simulink library "library"  (R2020b)
settings: Solver=VariableStepAuto  StartTime=0.0  StopTime=10.0  RelTol=1e-3
undefined symbols (not defined in the file): constants, orbit, sensors, spacecraft
libraries: vrlib x6, cstblocks x1, $bdroot x1
settings Model: Creator=loren  LastModifiedBy=loren

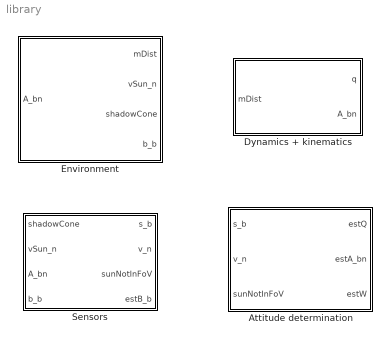
== system library ==
  Attitude determination : Subsystem
  Dynamics + kinematics : Subsystem
  Environment : Subsystem
  Sensors : Subsystem

== system library/Attitude determination ==
  s_b : Inport
  v_n : Inport  Port=2
  sunNotInFoV : Inport  Port=3
  Angular velocity estimation : Subsystem
  DCM : $bdroot/Kinematics/DCM  SystemSampleTime=-1  VariantActivationTime=update diagram  Latency=0  AutoFrameSizeCalculation=off
  MATLAB Function : MATLAB Function  TreatAsAtomicUnit=on
  Memory : Memory  InitialCondition=spacecraft.q0
  estQ : Outport
  estA_bn : Outport  Port=2
  estW : Outport  Port=3
  wires:
  s_b/1 -> MATLAB Function/1(s_b)
  v_n/1 -> MATLAB Function/2(v_n)
  sunNotInFoV/1 -> MATLAB Function/3(sunNotInFoV)
  DCM/1 -> estA_bn/1
  Angular velocity estimation/1(estW) -> estW/1
  MATLAB Function/1(estQ) -> Memory/1, estQ/1, DCM/1, Angular velocity estimation/1(estQ)
  Memory/1 -> MATLAB Function/4(q_old)

== system library/Dynamics + kinematics ==
  mDist : Inport
  Euler eqns. : Subsystem
  Kinematics : Subsystem
  q : Outport
  A_bn : Outport  Port=2
  wires:
  mDist/1 -> Euler eqns./1(mDist)
  Euler eqns./1(w) -> Kinematics/1(w)
  Kinematics/1(q) -> q/1
  Kinematics/2(A_bn) -> A_bn/1

== system library/Environment ==
  A_bn : Inport
  Disturbances : Subsystem
  Orbit propagator : Subsystem
  mDist : Outport
  vSun_n : Outport  Port=2
  shadowCone : Outport  Port=3
  b_b : Outport  Port=4
  wires:
  A_bn/1 -> Disturbances/3(A_bn), Orbit propagator/1(A_bn)
  Orbit propagator/1(rrSc_n) -> Disturbances/1(rrSc_n)
  Orbit propagator/2(vvSc_n) -> Disturbances/2(vvSc_n)
  Orbit propagator/3(A_bl) -> Disturbances/4(A_bl)
  Disturbances/1(mDist) -> mDist/1
  Disturbances/2(vSun_n) -> vSun_n/1
  Disturbances/3(shadowCone) -> shadowCone/1
  Disturbances/4(b_b) -> b_b/1

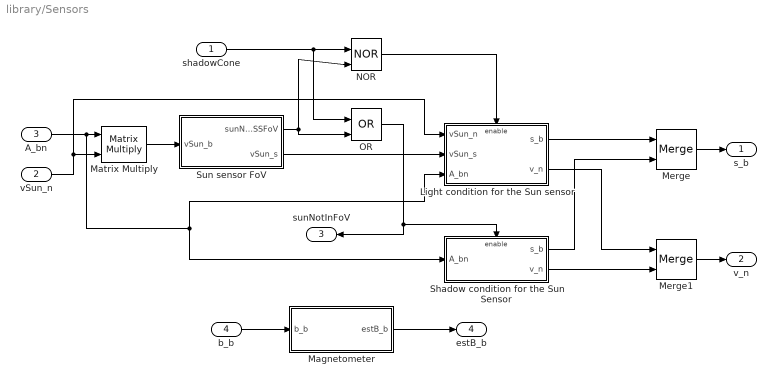
== system library/Sensors ==
  shadowCone : Inport
  vSun_n : Inport  Port=2
  A_bn : Inport  Port=3
  b_b : Inport  Port=4
  Light condition for the Sun sensor : Subsystem  TreatAsAtomicUnit=on
  Magnetometer : Subsystem
  Matrix Multiply : Product  Multiplication=Matrix(*)
  Merge : Merge
  Merge1 : Merge
  NOR : Logic  Operator=NOR  IconShape=distinctive  AllPortsSameDT=off  OutDataTypeStr=boolean
  OR : Logic  Operator=OR  IconShape=distinctive  AllPortsSameDT=off  OutDataTypeStr=boolean
  Shadow condition for the Sun Sensor : Subsystem  TreatAsAtomicUnit=on
  Sun sensor FoV : Subsystem
  s_b : Outport
  v_n : Outport  Port=2
  sunNotInFoV : Outport  Port=3
  estB_b : Outport  Port=4
  wires:
  Sun sensor FoV/1(sunNotInSSFoV) -> OR/2, NOR/2
  shadowCone/1 -> NOR/1, OR/1
  Matrix Multiply/1 -> Sun sensor FoV/1(vSun_b)
  vSun_n/1 -> Light condition for the Sun sensor/1(vSun_n), Matrix Multiply/2
  A_bn/1 -> Shadow condition for the Sun Sensor/1(A_bn), Light condition for the Sun sensor/3(A_bn), Matrix Multiply/1
  Merge/1 -> s_b/1
  Merge1/1 -> v_n/1
  OR/1 -> Shadow condition for the Sun Sensor/Enable, sunNotInFoV/1
  Sun sensor FoV/2(vSun_s) -> Light condition for the Sun sensor/2(vSun_s)
  Light condition for the Sun sensor/1(s_b) -> Merge/1
  Shadow condition for the Sun Sensor/1(s_b) -> Merge/2
  Shadow condition for the Sun Sensor/2(v_n) -> Merge1/2
  Light condition for the Sun sensor/2(v_n) -> Merge1/1
  NOR/1 -> Light condition for the Sun sensor/Enable
  b_b/1 -> Magnetometer/1(b_b)
  Magnetometer/1(estB_b) -> estB_b/1

== system library/Attitude determination/Angular velocity estimation ==
  estQ : Inport
  Constant : Constant
  Derivative : Derivative  CoefficientInTFapproximation=1/100
  Gain : Gain  Gain=2
  MATLAB Function : MATLAB Function  TreatAsAtomicUnit=on
  Matrix Multiply : Product  Multiplication=Matrix(*)
  Varying Lowpass Filter : cstblocks/Linear Parameter Varying/Varying Lowpass Filter  N=2
  estW : Outport
  wires:
  estQ/1 -> Varying Lowpass Filter/1, MATLAB Function/1(q)
  MATLAB Function/1(pinvQ) -> Matrix Multiply/1
  Derivative/1 -> Matrix Multiply/2  "dotQest"
  Matrix Multiply/1 -> Gain/1
  Gain/1 -> estW/1
  Varying Lowpass Filter/1 -> Derivative/1
  Constant/1 -> Varying Lowpass Filter/2

== system library/Dynamics + kinematics/Euler eqns. ==
  mDist : Inport
  Add : Sum  Inputs=-+
  Constant : Constant  Value=spacecraft.I
  Cross Product : vrlib/Utilities/Cross Product
  Gain : Gain  Gain=spacecraft.invI  Multiplication=Matrix(K*u) (u vector)
  Integrator : Integrator  InitialCondition=spacecraft.w0
  Product : Product  Multiplication=Matrix(*)
  w : Outport
  wires:
  Constant/1 -> Product/1
  Integrator/1 -> w/1, Product/2, Cross Product/2  "w"
  Product/1 -> Cross Product/1
  mDist/1 -> Add/2
  Cross Product/1 -> Add/1
  Add/1 -> Gain/1
  Gain/1 -> Integrator/1

== system library/Dynamics + kinematics/Kinematics ==
  w : Inport
  DCM : Subsystem
  Quaternion integration : Subsystem
  q : Outport
  A_bn : Outport  Port=2
  wires:
  w/1 -> Quaternion integration/1(w)
  Quaternion integration/1(q) -> q/1, DCM/1(q)
  DCM/1(A_bn) -> A_bn/1

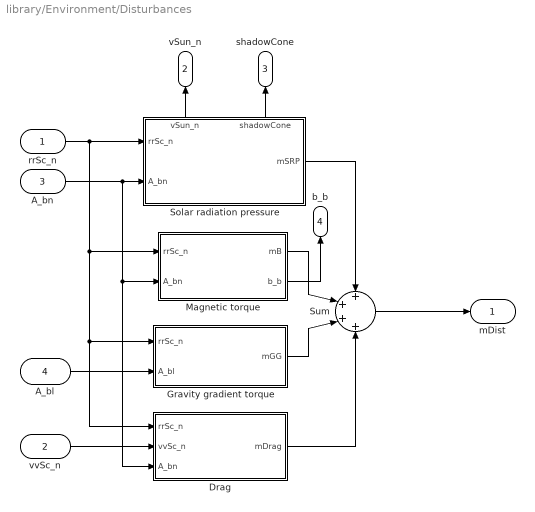
== system library/Environment/Disturbances ==
  rrSc_n : Inport
  vvSc_n : Inport  Port=2
  A_bn : Inport  Port=3
  A_bl : Inport  Port=4
  Drag : Subsystem
  Gravity gradient torque : Subsystem
  Magnetic torque : Subsystem
  Solar radiation pressure : Subsystem
      settings: PortSchema="{\"entries\":[{\"content\":{\"sides\":[{\"content\":{\"connectorIds\":[\"In1\",\"In2\"]},\"type\":\"ConnectorPlacement.EquallySpacedRectSide\",\"uuid\":\"1c58e148-737e-4c26-8467-bf4a1427bac3\"},{\"content\":{\"connectorIds\":[\"Out1\"],\"side\":\"RIGHT\"},\"type\":\"ConnectorPlacement.EquallySpacedRectSide\",\"uuid\":\"1132a1c1-392d-4550-8b40-4ae647f3a6c1\"},{\"content\":{\"connectorIds\":[\"Out2\",\"Out3\"],\"side\":\"TOP\"},\"type\":\"ConnectorPlacement.EquallySpacedRectSide\",\"uuid\":\"8cec875a-7b2b-408d-843f-f50e353248f2\"},{\"content\":{\"connectorIds\":[],\"side\":\"HIDDEN\"},\"type\":\"ConnectorPlacement.EquallySpacedRectSide\",\"uuid\":\"95559ba3-4215-4144-a5e7-008848b1ca72\"}]},\"type\":\"ConnectorPlacement.EquallySpacedConnector\",\"uuid\":\"cb15f690-b6d7-424c-84c7-df23a46a4e4f\"}],\"packageUris\":[\"http://schema.mathworks.com/mf0/Connector/R2020b\"],\"version\":\"1.0\"}"
  Sum : Sum  Inputs=++++
  mDist : Outport
  vSun_n : Outport  Port=2
  shadowCone : Outport  Port=3
  b_b : Outport  Port=4
  wires:
  Solar radiation pressure/1(mSRP) -> Sum/1
  A_bn/1 -> Drag/3(A_bn), Magnetic torque/2(A_bn), Solar radiation pressure/2(A_bn)
  vvSc_n/1 -> Drag/2(vvSc_n)
  rrSc_n/1 -> Gravity gradient torque/1(rrSc_n), Drag/1(rrSc_n), Magnetic torque/1(rrSc_n), Solar radiation pressure/1(rrSc_n)
  Gravity gradient torque/1(mGG) -> Sum/3
  Drag/1(mDrag) -> Sum/4
  Magnetic torque/1(mB) -> Sum/2
  Sum/1 -> mDist/1
  A_bl/1 -> Gravity gradient torque/2(A_bl)
  Solar radiation pressure/2(vSun_n) -> vSun_n/1
  Solar radiation pressure/3(shadowCone) -> shadowCone/1
  Magnetic torque/2(b_b) -> b_b/1

== system library/Environment/Orbit propagator ==
  A_bn : Inport
  Integrator : Integrator  InitialCondition=orbit.theta0
  LVLH frame : Subsystem
  Position and velocity (inertial frame) : Subsystem
  True anomaly ODE : Subsystem
  rrSc_n : Outport
  vvSc_n : Outport  Port=2
  A_bl : Outport  Port=3
  wires:
  True anomaly ODE/1(theta_dot) -> Integrator/1
  Integrator/1 -> True anomaly ODE/1(theta), Position and velocity (inertial frame)/1(theta), LVLH frame/1(theta)
  Position and velocity (inertial frame)/1(rrSc_n) -> rrSc_n/1
  Position and velocity (inertial frame)/2(vvSc_n) -> vvSc_n/1
  LVLH frame/1(A_bl) -> A_bl/1
  A_bn/1 -> LVLH frame/2(A_bn)

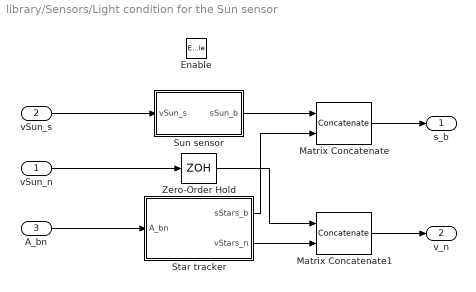
== system library/Sensors/Light condition for the Sun sensor ==
  vSun_n : Inport
  vSun_s : Inport  Port=2
  A_bn : Inport  Port=3
  Enable : EnablePort
  Matrix Concatenate : Concatenate  Mode=Multidimensional array  ConcatenateDimension=2
  Matrix Concatenate1 : Concatenate  Mode=Multidimensional array  ConcatenateDimension=2
  Star tracker : Subsystem
  Sun sensor : Subsystem
  Zero-Order Hold : ZeroOrderHold  SampleTime=max([sensors.ss.Ts, sensors.st.Ts])
  s_b : Outport
  v_n : Outport  Port=2
  wires:
  vSun_s/1 -> Sun sensor/1(vSun_s)
  A_bn/1 -> Star tracker/1(A_bn)
  Sun sensor/1(sSun_b) -> Matrix Concatenate/1
  Star tracker/1(sStars_b) -> Matrix Concatenate/2
  Star tracker/2(vStars_n) -> Matrix Concatenate1/2
  vSun_n/1 -> Zero-Order Hold/1
  Matrix Concatenate/1 -> s_b/1
  Matrix Concatenate1/1 -> v_n/1
  Zero-Order Hold/1 -> Matrix Concatenate1/1

== system library/Sensors/Magnetometer ==
  b_b : Inport
  Add : Sum
  MATLAB Function : MATLAB Function  TreatAsAtomicUnit=on
  Matrix Multiply : Product  Multiplication=Matrix(*)
  Random Number : RandomNumber  Variance=sensors.mm.sigmaPhi^2  Seed=randi(1e5, 1, 1)  SampleTime=sensors.mm.Ts
  Random Number1 : RandomNumber  Variance=sensors.mm.sigmaTheta^2  Seed=randi(1e5, 1, 1)  SampleTime=sensors.mm.Ts
  Random Number2 : RandomNumber  Variance=sensors.mm.sigmaPsi^2  Seed=randi(1e5, 1, 1)  SampleTime=sensors.mm.Ts
  Random Number3 : RandomNumber  Variance=sensors.mm.eps^2*ones(3,1)  Seed=randi(1e5, 1, 1)  SampleTime=sensors.mm.Ts
  Zero-Order Hold : ZeroOrderHold  SampleTime=sensors.mm.Ts
  estB_b : Outport
  wires:
  b_b/1 -> Zero-Order Hold/1
  Random Number/1 -> MATLAB Function/1(phi)
  Random Number1/1 -> MATLAB Function/2(theta)
  Random Number2/1 -> MATLAB Function/3(psi)
  Zero-Order Hold/1 -> Add/1
  MATLAB Function/1(A_err) -> Matrix Multiply/1
  Matrix Multiply/1 -> estB_b/1
  Add/1 -> Matrix Multiply/2
  Random Number3/1 -> Add/2

== system library/Sensors/Shadow condition for the Sun Sensor ==
  A_bn : Inport
  Enable : EnablePort
  Star tracker : Subsystem
  s_b : Outport
  v_n : Outport  Port=2
  wires:
  Star tracker/1(sStars_b) -> s_b/1
  Star tracker/2(vStars_n) -> v_n/1
  A_bn/1 -> Star tracker/1(A_bn)

== system library/Sensors/Sun sensor FoV ==
  vSun_b : Inport
  Acos : Trigonometry  Operator=acos
  Constant : Constant  Value=sensors.ss.FoV/2
  Constant1 : Constant  Value=sensors.ss.A_sb
  Dot Product : DotProduct  InputSameDT=on  OutDataTypeStr=Inherit: Inherit via internal rule
  Gain : Gain  Gain=sensors.ss.A_sb  Multiplication=Matrix(K*u) (u vector)
  Less Than : RelationalOperator  Operator=>  OutDataTypeStr=boolean  RndMeth=Simplest
  Normalize Vector : vrlib/Utilities/Normalize Vector  maxzero=0
  Selector : Selector  NumberOfDimensions=2  InputPortWidth=3  IndexOptions=Index vector (dialog),Index vector (dialog)  Indices=[1 2 3],[1]  OutputSizes=1,1
  sunNotInSSFoV : Outport
  vSun_s : Outport  Port=2
  wires:
  Constant1/1 -> Selector/1
  Less Than/1 -> sunNotInSSFoV/1
  Constant/1 -> Less Than/2
  Acos/1 -> Less Than/1
  Dot Product/1 -> Acos/1
  vSun_b/1 -> Gain/1
  Normalize Vector/1 -> Dot Product/1
  Selector/1 -> Normalize Vector/1
  Gain/1 -> Dot Product/2, vSun_s/1

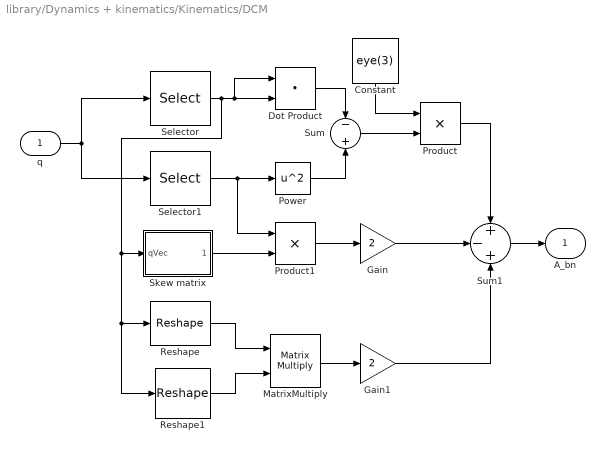
== system library/Dynamics + kinematics/Kinematics/DCM ==
  q : Inport
  Constant : Constant  Value=eye(3)
  Dot Product : DotProduct  InputSameDT=on  OutDataTypeStr=Inherit: Inherit via internal rule
  Gain : Gain  Gain=2
  Gain1 : Gain  Gain=2
  MatrixMultiply : Product  Multiplication=Matrix(*)
  Power : Math  Operator=square  SaturateOnIntegerOverflow=on
  Product : Product
  Product1 : Product
  Reshape : Reshape  OutputDimensionality=Column vector (2-D)
  Reshape1 : Reshape  OutputDimensionality=Row vector (2-D)
  Selector : Selector  InputPortWidth=4  IndexOptions=Index vector (dialog)  Indices=[1 2 3]  OutputSizes=1
  Selector1 : Selector  InputPortWidth=4  IndexOptions=Index vector (dialog)  Indices=[4]  OutputSizes=1
  Skew matrix : Subsystem
  Sum : Sum  Inputs=-+
  Sum1 : Sum  Inputs=+-+
  A_bn : Outport
  wires:
  q/1 -> Selector/1, Selector1/1
  Selector/1 -> Reshape1/1, Reshape/1, Skew matrix/1(qVec), Dot Product/2, Dot Product/1
  Selector1/1 -> Product1/1, Power/1
  Power/1 -> Sum/2
  Dot Product/1 -> Sum/1
  Constant/1 -> Product/1
  Sum/1 -> Product/2
  Skew matrix/1(qWedge) -> Product1/2
  Product1/1 -> Gain/1
  Reshape/1 -> MatrixMultiply/1
  Reshape1/1 -> MatrixMultiply/2
  MatrixMultiply/1 -> Gain1/1
  Product/1 -> Sum1/1
  Gain/1 -> Sum1/2
  Gain1/1 -> Sum1/3
  Sum1/1 -> A_bn/1

== system library/Dynamics + kinematics/Kinematics/Quaternion integration ==
  w : Inport
  Gain : Gain  Gain=1/2
  Integrator : Integrator  InitialCondition=spacecraft.q0
  MatrixMultiply : Product  Multiplication=Matrix(*)
  Normalize Vector : vrlib/Utilities/Normalize Vector  maxzero=0
  Omega matrix : Subsystem
  q : Outport
  wires:
  Integrator/1 -> Normalize Vector/1
  w/1 -> Omega matrix/1(w)
  Normalize Vector/1 -> MatrixMultiply/2, q/1
  Omega matrix/1(OM_mat) -> MatrixMultiply/1
  MatrixMultiply/1 -> Gain/1
  Gain/1 -> Integrator/1

== system library/Environment/Disturbances/Drag ==
  rrSc_n : Inport
  vvSc_n : Inport  Port=2
  A_bn : Inport  Port=3
  Constant : Constant  Value=constants.rho
  MATLAB Function : MATLAB Function  TreatAsAtomicUnit=on
  mDrag : Outport
  wires:
  rrSc_n/1 -> MATLAB Function/1(rrSc_n)
  MATLAB Function/1(mDrag) -> mDrag/1
  vvSc_n/1 -> MATLAB Function/2(vvSc_n)
  A_bn/1 -> MATLAB Function/3(A_bn)
  Constant/1 -> MATLAB Function/4(rho)

== system library/Environment/Disturbances/Gravity gradient torque ==
  rrSc_n : Inport
  A_bl : Inport  Port=2
  Constant : Constant  Value=[1 0 0]
  GG : Subsystem
  MatrixMultiply : Product  Multiplication=Matrix(*)
  mGG : Outport
  wires:
  Constant/1 -> MatrixMultiply/2
  MatrixMultiply/1 -> GG/2(c)  "c"
  A_bl/1 -> MatrixMultiply/1
  GG/1(mGG) -> mGG/1
  rrSc_n/1 -> GG/1(rrSc_n)

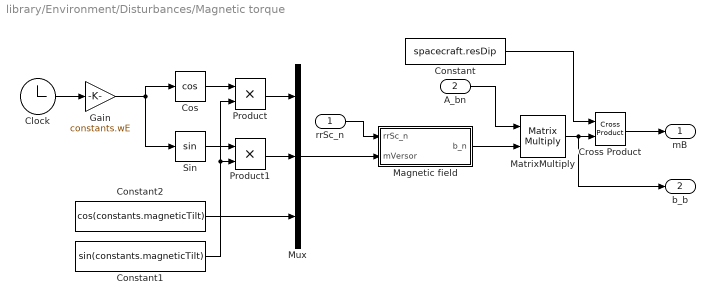
== system library/Environment/Disturbances/Magnetic torque ==
  rrSc_n : Inport
  A_bn : Inport  Port=2
  Clock : Clock
  Constant : Constant  Value=spacecraft.resDip
  Constant1 : Constant  Value=sin(constants.magneticTilt)
  Constant2 : Constant  Value=cos(constants.magneticTilt)
  Cos : Trigonometry  Operator=cos
  Cross Product : vrlib/Utilities/Cross Product
  Gain : Gain  Gain=constants.wE
  Magnetic field : Subsystem
  MatrixMultiply : Product  Multiplication=Matrix(*)
  Mux : Mux  Inputs=3
  Product : Product
  Product1 : Product
  Sin : Trigonometry
  mB : Outport
  b_b : Outport  Port=2
  wires:
  Clock/1 -> Gain/1
  Constant/1 -> Cross Product/1
  Gain/1 -> Sin/1, Cos/1
  Constant2/1 -> Mux/3
  Sin/1 -> Product1/1
  Cos/1 -> Product/1
  Product/1 -> Mux/1
  Product1/1 -> Mux/2
  Constant1/1 -> Product/2, Product1/2
  A_bn/1 -> MatrixMultiply/1
  rrSc_n/1 -> Magnetic field/1(rrSc_n)
  Mux/1 -> Magnetic field/2(mVersor)
  Magnetic field/1(b_n) -> MatrixMultiply/2
  MatrixMultiply/1 -> b_b/1, Cross Product/2
  Cross Product/1 -> mB/1

== system library/Environment/Disturbances/Solar radiation pressure ==
  note: Determine whether the s/c is in sunlight or not
  rrSc_n : Inport
  A_bn : Inport  Port=2
  If : If  IfExpression=u1 == 1
  If Action Subsystem : Subsystem  TreatAsAtomicUnit=on
  If Action Subsystem1 : Subsystem  TreatAsAtomicUnit=on
  MATLAB Function2 : MATLAB Function  TreatAsAtomicUnit=on
  Merge1 : Merge
  Sun position in Earth inertial frame : Subsystem
  mSRP : Outport
  vSun_n : Outport  Port=2
  shadowCone : Outport  Port=3
  wires:
  MATLAB Function2/1(shadowCone) -> shadowCone/1, If/1
  If/2 -> If Action Subsystem/Action
  If/1 -> If Action Subsystem1/Action
  If Action Subsystem/1(mSRP) -> Merge1/2
  rrSc_n/1 -> If Action Subsystem1/1(rrSc_n), MATLAB Function2/1(rrSc_n)
  Merge1/1 -> mSRP/1
  If Action Subsystem1/1(mSRP) -> Merge1/1
  A_bn/1 -> If Action Subsystem1/3(A_bn)
  Sun position in Earth inertial frame/1(rrSun_n) -> If Action Subsystem1/2(rrSun_n), MATLAB Function2/2(rrSun_n)
  If Action Subsystem1/2(vSun_n) -> vSun_n/1

== system library/Environment/Orbit propagator/LVLH frame ==
  theta : Inport
  A_bn : Inport  Port=2
  LVLH to inclined orbit frame : Subsystem
  Product : Product  Multiplication=Matrix(*)
  Product1 : Product  Multiplication=Matrix(*)
  R1(i) : Constant  Value=[1 0 0; 0 cos(orbit.i) sin(orbit.i); 0 -sin(orbit.i) cos(orbit.i)];
  Transpose : Math  Operator=transpose  SaturateOnIntegerOverflow=on
  A_bl : Outport
  wires:
  Transpose/1 -> Product1/2  "A_nl"
  Product/1 -> Transpose/1
  A_bn/1 -> Product1/1
  Product1/1 -> A_bl/1  "A_bl"
  R1(i)/1 -> Product/2
  theta/1 -> LVLH to inclined orbit frame/1(theta)
  LVLH to inclined orbit frame/1(A_li) -> Product/1

== system library/Environment/Orbit propagator/Position and velocity (inertial frame) ==
  theta : Inport
  MatrixMultiply : Product  Multiplication=Matrix(*)
  MatrixMultiply1 : Product  Multiplication=Matrix(*)
  Position and velocity (perifocal frame) : Subsystem
  R1(i) : Constant  Value=[1 0 0; 0 cos(orbit.i) sin(orbit.i); 0 -sin(orbit.i) cos(orbit.i)];
  R3(OM) : Constant  Value=[cos(orbit.OM), sin(orbit.OM), 0; -sin(orbit.OM), cos(orbit.OM), 0; 0, 0, 1]
  R3(om) : Constant  Value=[cos(orbit.om), sin(orbit.om), 0; -sin(orbit.om), cos(orbit.om), 0; 0, 0, 1]
  Rotation matrix (perifocal-inertial) : Product  Inputs=3  Multiplication=Matrix(*)
  Transpose : Math  Operator=transpose  SaturateOnIntegerOverflow=on
  rrSc_n : Outport
  vvSc_n : Outport  Port=2
  wires:
  MatrixMultiply/1 -> rrSc_n/1
  Position and velocity (perifocal frame)/2(vvSc_pf) -> MatrixMultiply1/2
  MatrixMultiply1/1 -> vvSc_n/1
  R3(om)/1 -> Rotation matrix (perifocal-inertial)/1
  R1(i)/1 -> Rotation matrix (perifocal-inertial)/2
  Rotation matrix (perifocal-inertial)/1 -> Transpose/1
  Transpose/1 -> MatrixMultiply1/1, MatrixMultiply/1
  R3(OM)/1 -> Rotation matrix (perifocal-inertial)/3
  Position and velocity (perifocal frame)/1(rrSc_pf) -> MatrixMultiply/2
  theta/1 -> Position and velocity (perifocal frame)/1(theta)

== system library/Environment/Orbit propagator/True anomaly ODE ==
  theta : Inport
  Add : Sum
  Constant1 : Constant
  Cos : Trigonometry  Operator=cos
  Gain : Gain  Gain=sqrt(constants.mu/orbit.a^3)
  Gain1 : Gain  Gain=(1 - orbit.e^2)^(-3/2)
  Gain2 : Gain  Gain=orbit.e
  Power : Math  Operator=square  SaturateOnIntegerOverflow=on
  theta_dot : Outport
  wires:
  theta/1 -> Cos/1
  Constant1/1 -> Add/1
  Cos/1 -> Gain2/1
  Gain2/1 -> Add/2
  Add/1 -> Power/1
  Power/1 -> Gain/1
  Gain/1 -> Gain1/1
  Gain1/1 -> theta_dot/1

== system library/Sensors/Light condition for the Sun sensor/Star tracker ==
  A_bn : Inport
  MATLAB Function : MATLAB Function  TreatAsAtomicUnit=on
  Memory : Memory  InitialCondition=sensors.st.vStars_n_init(:,2:end)  InheritSampleTime=on  LinearizeMemory=on
  Random Number : RandomNumber  Variance=sensors.st.sigmaPhi^2  Seed=randi(1e5,1,1)  SampleTime=max([sensors.ss.Ts, sensors.st.Ts])
  Random Number1 : RandomNumber  Variance=sensors.st.sigmaTheta^2  Seed=randi(1e5,1,1)  SampleTime=max([sensors.ss.Ts, sensors.st.Ts])
  Random Number2 : RandomNumber  Variance=sensors.st.sigmaPsi^2  Seed=randi(1e5,1,1)  SampleTime=max([sensors.ss.Ts, sensors.st.Ts])
  Zero-Order Hold : ZeroOrderHold  SampleTime=max([sensors.ss.Ts, sensors.st.Ts])
  sStars_b : Outport
  vStars_n : Outport  Port=2
  wires:
  MATLAB Function/2(v_n) -> Memory/1, vStars_n/1
  MATLAB Function/1(s_b) -> sStars_b/1
  Random Number1/1 -> MATLAB Function/3(theta)
  A_bn/1 -> Zero-Order Hold/1
  Random Number2/1 -> MATLAB Function/4(psi)
  Random Number/1 -> MATLAB Function/2(phi)
  Zero-Order Hold/1 -> MATLAB Function/1(A_bn)
  Memory/1 -> MATLAB Function/5(v_n_old)

== system library/Sensors/Light condition for the Sun sensor/Sun sensor ==
  vSun_s : Inport
  MATLAB Function : MATLAB Function  TreatAsAtomicUnit=on
  MatrixMultiply1 : Product  Multiplication=Matrix(*)
  Random Number : RandomNumber  Variance=sensors.ss.sigmaPhi^2  Seed=randi(1e5, 1, 1)  SampleTime=max([sensors.ss.Ts, sensors.st.Ts])
  Random Number1 : RandomNumber  Variance=sensors.ss.sigmaTheta^2  Seed=randi(1e5, 1, 1)  SampleTime=max([sensors.ss.Ts, sensors.st.Ts])
  Random Number2 : RandomNumber  Variance=sensors.ss.sigmaPsi^2  Seed=randi(1e5, 1, 1)  SampleTime=max([sensors.ss.Ts, sensors.st.Ts])
  Zero-Order Hold : ZeroOrderHold  SampleTime=max([sensors.ss.Ts, sensors.st.Ts])
  sSun_b : Outport
  wires:
  Random Number/1 -> MATLAB Function/1(phi)
  Random Number1/1 -> MATLAB Function/2(theta)
  MATLAB Function/1(A_err) -> MatrixMultiply1/1
  MatrixMultiply1/1 -> sSun_b/1
  Random Number2/1 -> MATLAB Function/3(psi)
  vSun_s/1 -> Zero-Order Hold/1  "vSun_s"
  Zero-Order Hold/1 -> MatrixMultiply1/2

== system library/Sensors/Shadow condition for the Sun Sensor/Star tracker ==
  A_bn : Inport
  MATLAB Function : MATLAB Function  TreatAsAtomicUnit=on
  Memory : Memory  InitialCondition=sensors.st.vStars_n_init  InheritSampleTime=on  LinearizeMemory=on
  Random Number : RandomNumber  Variance=sensors.st.sigmaPhi^2  Seed=randi(1e5,1,1)  SampleTime=max([sensors.ss.Ts, sensors.st.Ts])
  Random Number1 : RandomNumber  Variance=sensors.st.sigmaTheta^2  Seed=randi(1e5,1,1)  SampleTime=max([sensors.ss.Ts, sensors.st.Ts])
  Random Number2 : RandomNumber  Variance=sensors.st.sigmaPsi^2  Seed=randi(1e5,1,1)  SampleTime=max([sensors.ss.Ts, sensors.st.Ts])
  Zero-Order Hold : ZeroOrderHold  SampleTime=max([sensors.ss.Ts, sensors.st.Ts])
  sStars_b : Outport
  vStars_n : Outport  Port=2
  wires:
  Memory/1 -> MATLAB Function/5(v_n_old)
  Zero-Order Hold/1 -> MATLAB Function/1(A_bn)
  Random Number/1 -> MATLAB Function/2(phi)
  Random Number2/1 -> MATLAB Function/4(psi)
  A_bn/1 -> Zero-Order Hold/1
  Random Number1/1 -> MATLAB Function/3(theta)
  MATLAB Function/1(s_b) -> sStars_b/1
  MATLAB Function/2(v_n) -> Memory/1, vStars_n/1

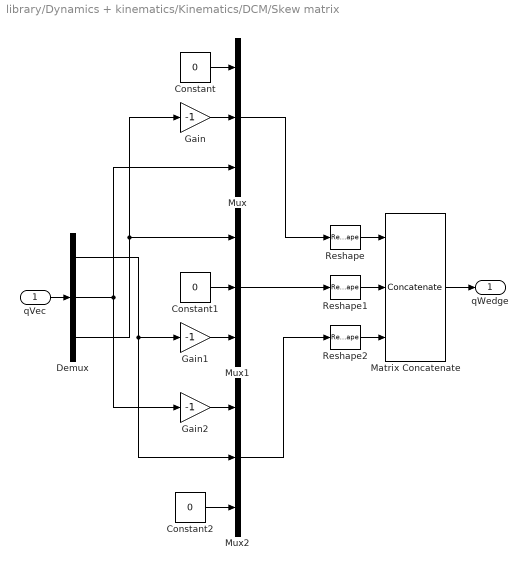
== system library/Dynamics + kinematics/Kinematics/DCM/Skew matrix ==
  qVec : Inport
  Constant : Constant  Value=0
  Constant1 : Constant  Value=0
  Constant2 : Constant  Value=0
  Demux : Demux  Outputs=3
  Gain : Gain  Gain=-1
  Gain1 : Gain  Gain=-1
  Gain2 : Gain  Gain=-1
  Matrix Concatenate : Concatenate  NumInputs=3  Mode=Multidimensional array
  Mux : Mux  Inputs=3
  Mux1 : Mux  Inputs=3
  Mux2 : Mux  Inputs=3
  Reshape : Reshape  OutputDimensionality=Row vector (2-D)
  Reshape1 : Reshape  OutputDimensionality=Row vector (2-D)
  Reshape2 : Reshape  OutputDimensionality=Row vector (2-D)
  qWedge : Outport
  wires:
  qVec/1 -> Demux/1
  Constant/1 -> Mux/1
  Gain/1 -> Mux/2
  Demux/3 -> Mux1/1, Gain/1
  Demux/2 -> Gain2/1, Mux/3
  Constant1/1 -> Mux1/2
  Gain1/1 -> Mux1/3
  Demux/1 -> Mux2/2, Gain1/1
  Constant2/1 -> Mux2/3
  Gain2/1 -> Mux2/1
  Mux1/1 -> Reshape1/1
  Mux/1 -> Reshape/1
  Mux2/1 -> Reshape2/1
  Matrix Concatenate/1 -> qWedge/1
  Reshape/1 -> Matrix Concatenate/1
  Reshape1/1 -> Matrix Concatenate/2
  Reshape2/1 -> Matrix Concatenate/3

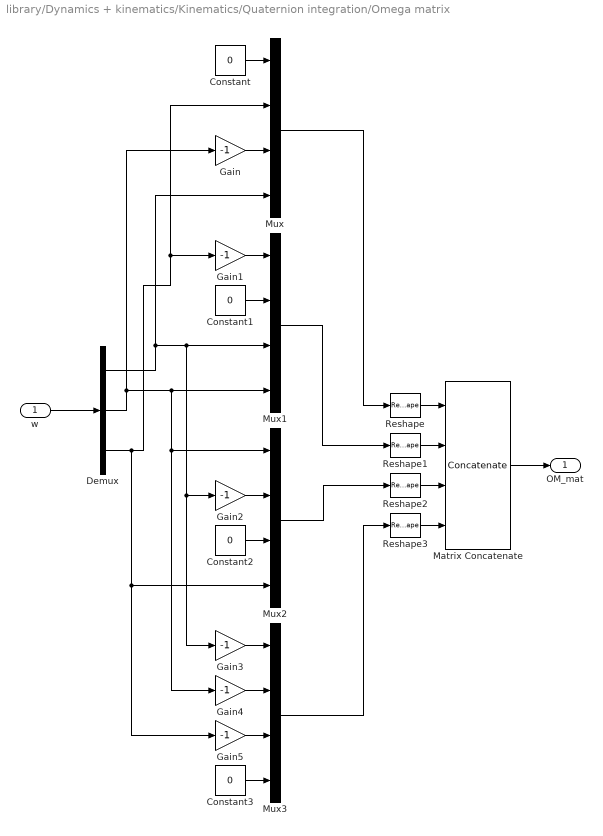
== system library/Dynamics + kinematics/Kinematics/Quaternion integration/Omega matrix ==
  w : Inport
  Constant{,1..3} (4 alike) : Constant  Value=0
  Demux : Demux  Outputs=3
  Gain{,1..5} (6 alike) : Gain  Gain=-1
  Matrix Concatenate : Concatenate  NumInputs=4  Mode=Multidimensional array
  Mux{,1..3} (4 alike) : Mux
  Reshape{,1..3} (4 alike) : Reshape  OutputDimensionality=Row vector (2-D)
  OM_mat : Outport
  wires:
  w/1 -> Demux/1
  Demux/1 -> Mux/4, Gain3/1, Gain2/1, Mux1/3
  Demux/2 -> Gain/1, Mux2/1, Gain4/1, Mux1/4
  Gain/1 -> Mux/3
  Demux/3 -> Mux/2, Gain1/1, Mux2/4, Gain5/1
  Constant/1 -> Mux/1
  Gain1/1 -> Mux1/1
  Constant1/1 -> Mux1/2
  Gain2/1 -> Mux2/2
  Constant2/1 -> Mux2/3
  Gain3/1 -> Mux3/1
  Gain4/1 -> Mux3/2
  Constant3/1 -> Mux3/4
  Gain5/1 -> Mux3/3
  Mux/1 -> Reshape/1
  Mux1/1 -> Reshape1/1
  Mux2/1 -> Reshape2/1
  Mux3/1 -> Reshape3/1
  Matrix Concatenate/1 -> OM_mat/1
  Reshape/1 -> Matrix Concatenate/1
  Reshape1/1 -> Matrix Concatenate/2
  Reshape2/1 -> Matrix Concatenate/3
  Reshape3/1 -> Matrix Concatenate/4

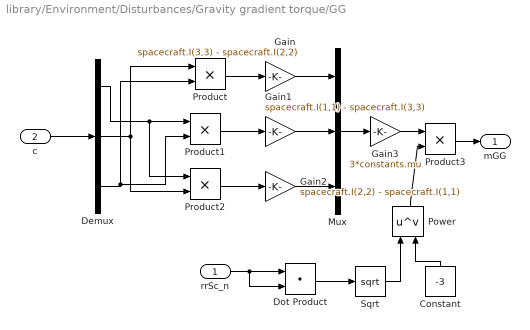
== system library/Environment/Disturbances/Gravity gradient torque/GG ==
  rrSc_n : Inport
  c : Inport  Port=2
  Constant : Constant  Value=-3
  Demux : Demux  Outputs=3
  Dot Product : DotProduct  InputSameDT=on  OutDataTypeStr=Inherit: Inherit via internal rule
  Gain : Gain  Gain=spacecraft.I(3,3) - spacecraft.I(2,2)
  Gain1 : Gain  Gain=spacecraft.I(1,1) - spacecraft.I(3,3)
  Gain2 : Gain  Gain=spacecraft.I(2,2) - spacecraft.I(1,1)
  Gain3 : Gain  Gain=3*constants.mu
  Mux : Mux  Inputs=3
  Power : Math  Operator=pow  SaturateOnIntegerOverflow=on
  Product{,1..3} (4 alike) : Product
  Sqrt : Sqrt  SaturateOnIntegerOverflow=on
  mGG : Outport
  wires:
  c/1 -> Demux/1
  Product/1 -> Gain/1
  Product1/1 -> Gain1/1
  Product2/1 -> Gain2/1
  Demux/2 -> Product2/2, Product/1
  Demux/3 -> Product1/2, Product/2
  Demux/1 -> Product2/1, Product1/1
  Gain2/1 -> Mux/3
  Gain1/1 -> Mux/2
  Gain/1 -> Mux/1
  Mux/1 -> Gain3/1
  Gain3/1 -> Product3/1
  Product3/1 -> mGG/1
  rrSc_n/1 -> Dot Product/2, Dot Product/1
  Dot Product/1 -> Sqrt/1
  Sqrt/1 -> Power/1
  Power/1 -> Product3/2
  Constant/1 -> Power/2

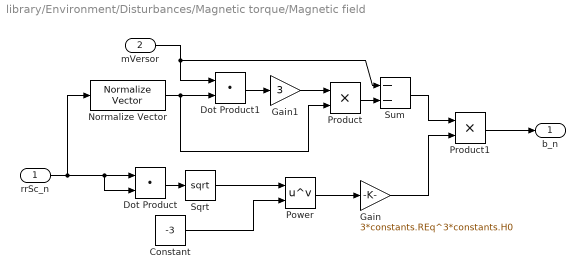
== system library/Environment/Disturbances/Magnetic torque/Magnetic field ==
  rrSc_n : Inport
  mVersor : Inport  Port=2
  Constant : Constant  Value=-3
  Dot Product : DotProduct  InputSameDT=on  OutDataTypeStr=Inherit: Inherit via internal rule
  Dot Product1 : DotProduct  InputSameDT=on  OutDataTypeStr=Inherit: Inherit via internal rule
  Gain : Gain  Gain=3*constants.REq^3*constants.H0
  Gain1 : Gain  Gain=3
  Normalize Vector : vrlib/Utilities/Normalize Vector  maxzero=0
  Power : Math  Operator=pow  SaturateOnIntegerOverflow=on
  Product : Product
  Product1 : Product
  Sqrt : Sqrt  SaturateOnIntegerOverflow=on
  Sum : Sum  Inputs=--
  b_n : Outport
  wires:
  rrSc_n/1 -> Normalize Vector/1, Dot Product/2, Dot Product/1
  Constant/1 -> Power/2
  Dot Product/1 -> Sqrt/1
  Sqrt/1 -> Power/1
  Power/1 -> Gain/1
  Normalize Vector/1 -> Product/2, Dot Product1/2
  mVersor/1 -> Sum/1, Dot Product1/1
  Dot Product1/1 -> Gain1/1
  Gain1/1 -> Product/1
  Product/1 -> Sum/2
  Sum/1 -> Product1/1
  Gain/1 -> Product1/2
  Product1/1 -> b_n/1

== system library/Environment/Disturbances/Solar radiation pressure/If Action Subsystem ==
  Action Port : ActionPort
  Constant1 : Constant  Value=[0;0;0]
  mSRP : Outport
  wires:
  Constant1/1 -> mSRP/1

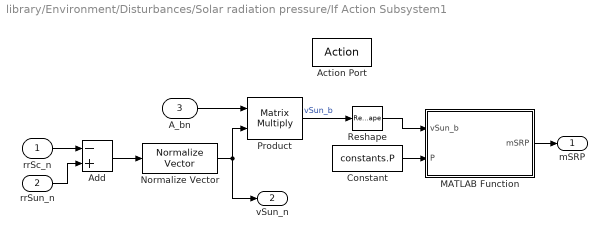
== system library/Environment/Disturbances/Solar radiation pressure/If Action Subsystem1 ==
  rrSc_n : Inport
  rrSun_n : Inport  Port=2
  A_bn : Inport  Port=3
  Action Port : ActionPort
  Add : Sum  Inputs=-+
  Constant : Constant  Value=constants.P
  MATLAB Function : MATLAB Function  TreatAsAtomicUnit=on
  Normalize Vector : vrlib/Utilities/Normalize Vector  maxzero=0
  Product : Product  Multiplication=Matrix(*)
  Reshape : Reshape  OutputDimensionality=Column vector (2-D)
  mSRP : Outport
  vSun_n : Outport  Port=2
  wires:
  A_bn/1 -> Product/1
  rrSun_n/1 -> Add/2
  Product/1 -> Reshape/1  "vSun_b"
  Normalize Vector/1 -> vSun_n/1, Product/2
  Add/1 -> Normalize Vector/1
  MATLAB Function/1(mSRP) -> mSRP/1
  rrSc_n/1 -> Add/1
  Constant/1 -> MATLAB Function/2(P)
  Reshape/1 -> MATLAB Function/1(vSun_b)

== system library/Environment/Disturbances/Solar radiation pressure/Sun position in Earth inertial frame ==
  Clock : Clock
  Cos : Trigonometry  Operator=cos
  Gain : Gain  Gain=constants.nSun
  Gain1 : Gain  Gain=cos(constants.oblAngle)
  Gain2 : Gain  Gain=sin(constants.oblAngle)
  Gain3 : Gain  Gain=1*constants.AU
  Mux : Mux  Inputs=3
  Sin1 : Trigonometry
  rrSun_n : Outport
  wires:
  Gain2/1 -> Mux/3
  Clock/1 -> Gain/1
  Gain/1 -> Sin1/1, Cos/1
  Gain1/1 -> Mux/2
  Mux/1 -> Gain3/1
  Sin1/1 -> Gain2/1, Gain1/1
  Cos/1 -> Mux/1
  Gain3/1 -> rrSun_n/1

== system library/Environment/Orbit propagator/LVLH frame/LVLH to inclined orbit frame ==
  theta : Inport
  Constant : Constant  Value=0
  Constant1 : Constant  Value=[0 0 1]
  Cos : Trigonometry  Operator=cos
  Gain : Gain  Gain=-1
  Mux : Mux  Inputs=3
  Mux1 : Mux  Inputs=3
  Sin : Trigonometry
  Vector Concatenate : Concatenate  NumInputs=3  Mode=Multidimensional array  ConcatenateDimension=2
  A_li : Outport
  wires:
  theta/1 -> Sin/1, Cos/1
  Cos/1 -> Mux1/2, Mux/1
  Sin/1 -> Gain/1, Mux/2
  Constant/1 -> Mux1/3, Mux/3
  Gain/1 -> Mux1/1
  Mux/1 -> Vector Concatenate/1
  Constant1/1 -> Vector Concatenate/3
  Mux1/1 -> Vector Concatenate/2
  Vector Concatenate/1 -> A_li/1

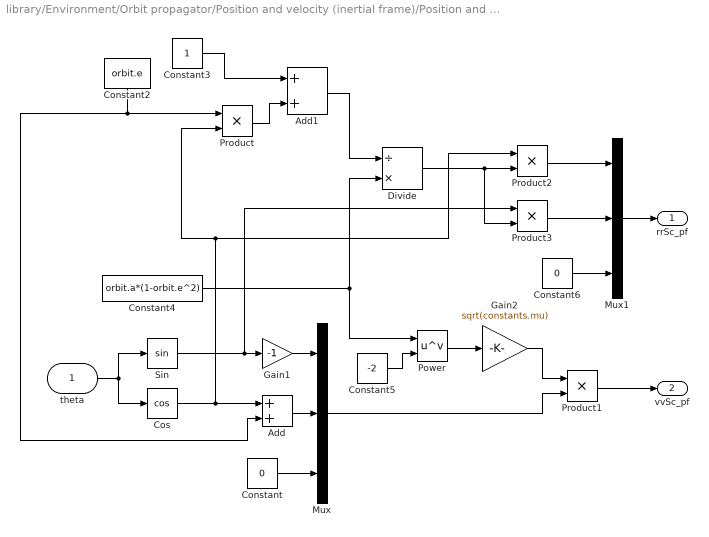
== system library/Environment/Orbit propagator/Position and velocity (inertial frame)/Position and velocity (perifocal frame) ==
  theta : Inport
  Add : Sum
  Add1 : Sum
  Constant : Constant  Value=0
  Constant2 : Constant  Value=orbit.e
  Constant3 : Constant
  Constant4 : Constant  Value=orbit.a*(1-orbit.e^2)
  Constant5 : Constant  Value=-2
  Constant6 : Constant  Value=0
  Cos : Trigonometry  Operator=cos
  Divide : Product  Inputs=/*
  Gain1 : Gain  Gain=-1
  Gain2 : Gain  Gain=sqrt(constants.mu)
  Mux : Mux  Inputs=3
  Mux1 : Mux  Inputs=3
  Power : Math  Operator=pow  SaturateOnIntegerOverflow=on
  Product{,1..3} (4 alike) : Product
  Sin : Trigonometry
  rrSc_pf : Outport
  vvSc_pf : Outport  Port=2
  wires:
  theta/1 -> Cos/1, Sin/1
  Mux/1 -> Product1/2
  Sin/1 -> Product3/1, Gain1/1
  Cos/1 -> Product2/1, Product/2, Add/1
  Gain1/1 -> Mux/1
  Add/1 -> Mux/2
  Constant/1 -> Mux/3
  Product1/1 -> vvSc_pf/1
  Constant3/1 -> Add1/1
  Constant2/1 -> Add/2, Product/1
  Product/1 -> Add1/2
  Add1/1 -> Divide/1
  Constant4/1 -> Divide/2, Power/1
  Constant5/1 -> Power/2
  Power/1 -> Gain2/1
  Gain2/1 -> Product1/1
  Divide/1 -> Product3/2, Product2/2
  Product2/1 -> Mux1/1
  Product3/1 -> Mux1/2
  Constant6/1 -> Mux1/3
  Mux1/1 -> rrSc_pf/1

== matlab function library/Sensors/Shadow condition for the Sun Sensor/Star tracker/MATLAB Function ==
  data: A_bn input; s_b output; phi input; theta input; psi input; v_n_old input; v_n output; sensors parameter
function [s_b, v_n] = starTracker(A_bn, phi, theta, psi, v_n_old, sensors)

A_sb = sensors.st.A_sb;
nStars = sensors.st.nStars;
FoV = sensors.st.FoV;

A_bs = A_sb';
A_ns = A_bn'*A_bs;

s_b = zeros(3,nStars); 
v_n = zeros(3,nStars);

El = zeros(nStars,1);
Az = zeros(nStars,1);

for k = 0:nStars-1
    
    s_b_old = A_bn*v_n_old(:,end-k);
    v_s_old = A_sb*s_b_old;
    
    El_old = asin(v_s_old(3));
    Az_old = acos(v_s_old(1)/cos(El_old));
    
    if v_s_old(2) <= 0
        El_old = 2*pi - El_old;
    end
    
    if abs(Az_old) > FoV(1)/2 || abs(El_old) > FoV(2)/2
        Az(end-k) = 0.2*FoV(1)*(-1 + 2*rand(1,1));
        El(end-k) = 0.2*FoV(2)*(-1 + 2*rand(1,1));
        v_s = [cos(El(end-k))*cos(Az(end-k));...
            cos(El(end-k))*sin(Az(end-k));...
            sin(El(end-k))];
        A_err = [cos(psi)*cos(theta), cos(psi)*sin(theta)*sin(phi) + sin(psi)*cos(phi),...
            -cos(psi)*sin(theta)*cos(phi) + sin(psi)*sin(phi);...
            -sin(psi)*cos(theta), -sin(psi)*sin(theta)*sin(phi) + cos(psi)*cos(phi),...
            sin(psi)*sin(theta)*cos(phi) + cos(psi)*sin(phi);...
            sin(theta), -cos(theta)*sin(phi), cos(theta)*cos(phi)];
    else
        A_err = eye(3);
        v_s = v_s_old;
    end
   
   s_s = A_err*v_s;
   s_bTemp = A_bs*s_s;
   s_b(1:3, end-k) = s_bTemp./norm(s_bTemp); 
   v_nTemp = A_ns*v_s;
   v_n(1:3,end-k) = v_nTemp;
   v_n(1:3, end-k) = v_nTemp./norm(v_nTemp);
   
end

end

== matlab function library/Attitude determination/Angular velocity estimation/MATLAB Function ==
  data: q input; pinvQ output
function pinvQ = quat_matrix(q)

q1 = q(1);
q2 = q(2);
q3 = q(3);
q4 = q(4);

Q = [q4, -q3, q2;...
    q3, q4, -q1;...
    -q2, q1, q4;...
    -q1, -q2, -q3];

pinvQ = pinv(Q);

end

== matlab function library/Sensors/Magnetometer/MATLAB Function ==
  data: phi input; A_err output; theta input; psi input
function A_err = error_matrix(phi, theta, psi)

A_err = [cos(psi)*cos(theta), cos(psi)*sin(theta)*sin(phi) + sin(psi)*cos(phi),...
    -cos(psi)*sin(theta)*cos(phi) + sin(psi)*sin(phi);...
    -sin(psi)*cos(theta), -sin(psi)*sin(theta)*sin(phi) + cos(psi)*cos(phi),...
    sin(psi)*sin(theta)*cos(phi) + cos(psi)*sin(phi);...
    sin(theta), -cos(theta)*sin(phi), cos(theta)*cos(phi)];
            
end

== matlab function library/Environment/Disturbances/Solar radiation pressure/If Action Subsystem1/MATLAB Function ==
  data: vSun_b input; P input; mSRP output; surfaces parameter
function mSRP = srp(vSun_b, P, surfaces)

rSurf = surfaces.rSurf;
n = surfaces.n;
A = surfaces.A;
rhoS = surfaces.rhoS;
rhoD = surfaces.rhoD;

mSRP = zeros(3,1);

for k = 1:size(rSurf,1)
    n_b = n(:,k);
    s_dot = dot(vSun_b, n_b);
    if s_dot > 0
        rhoS_temp = rhoS(k);
        Fsrp_i = - P*A(k)*s_dot.*((1-rhoS_temp).*vSun_b +...
            (2*rhoS_temp*s_dot + 2/3*rhoD(k)).*n_b);
        mSRP = mSRP + cross(rSurf(:,k), Fsrp_i);
    end
end

% aggiungere questione su "ombra"

end

== matlab function library/Environment/Disturbances/Drag/MATLAB Function ==
  data: rrSc_n input; mDrag output; vvSc_n input; A_bn input; rho input; surfaces parameter
function  mDrag = drag(rrSc_n, vvSc_n, A_bn, rho, surfaces)

rSurf = surfaces.rSurf;
n = surfaces.n;
A = surfaces.A;
cd = surfaces.cd;

wE = 7.2921150e-5; %[rad/s]
vvRel_n = [vvSc_n(1) + wE*rrSc_n(2); vvSc_n(2) - wE*rrSc_n(1); vvSc_n(3)];
vvRel_b = A_bn*vvRel_n;

vRel = norm(vvRel_n);
vRel_b = norm(vvRel_b);
vvVersor = vvRel_b/vRel_b;

c = -1/2*rho*cd*vRel^2.*vvVersor;

mDrag = zeros(3,1);

for k = 1:size(rSurf,1)
        n_dot = dot(n(:,k), vvVersor);
    if n_dot > 0
        A_cross = A(k)*n_dot;
        Fdrag_i = c*A_cross;
        mDrag = mDrag + cross(rSurf(:,k), Fdrag_i);
    end
end

end

== matlab function library/Environment/Disturbances/Solar radiation pressure/MATLAB Function2 ==
  data: rrSc_n input; shadowCone output; rrSun_n input
function shadowCone = cone(rrSc_n, rrSun_n)

% PROTOTYPE:
%  shadow_cone = cone(rr_sc, rr_sun_n)
% 
% DESCRIPTION:
%   This function returns a parameter that is 1 if the s/c is out of the 
%   planet's shadow cone (SRP effects considerable) or 0 if the s/c is 
%   inside the planet's shadow cone (NO SRP)
% 
% INPUT:
% rr_sc:            geocentric position vector of the s/c
% rr_sun_n:        geocentric position vector of the sun
%
% OUTPUT:
% shadow_cone:      boolean parameter (0 or 1)
%
% CONTRIBUTORS:
% Velo Giacomo
%
% VERSIONS:
% 2019-12-10 first version
%
% CALLED FUNCTIONS:
%     none


Req = 6378.1;
r = norm(rrSc_n);     
r_sun = norm(rrSun_n);
% Angle between s/c geocentric position and the tangent to Earth's surface
theta_sc = acos(Req/r);
% Angle between sun geocentric position and the tangent to Earth's surface
theta_sun = acos(Req/r_sun);
% Angle between s/c geocentric position and sun geocentric position
theta = acos(dot(rrSc_n, rrSun_n)/(r*r_sun));

% If the s/c is inside the shadow cone of the planet the value of
% shadow_cone will be = 0

    if theta_sc + theta_sun <= theta
        shadowCone = 0;
    else
        shadowCone = 1;
    end

end

== matlab function library/Sensors/Light condition for the Sun sensor/Star tracker/MATLAB Function ==
  data: A_bn input; s_b output; phi input; theta input; psi input; v_n_old input; v_n output; sensors parameter
function [s_b, v_n] = starTracker(A_bn, phi, theta, psi, v_n_old, sensors)

A_sb = sensors.st.A_sb;
nStars = sensors.st.nStars - 1;
FoV = sensors.st.FoV;

A_bs = A_sb';
A_ns = A_bn'*A_bs;

s_b = zeros(3,nStars); 
v_n = zeros(3,nStars);

El = zeros(nStars,1);
Az = zeros(nStars,1);

for k = 0:nStars-1
    
    s_b_old = A_bn*v_n_old(:,end-k);
    v_s_old = A_sb*s_b_old;
    
    El_old = asin(v_s_old(3));
    Az_old = acos(v_s_old(1)/cos(El_old));
    
    if v_s_old(2) <= 0
        El_old = 2*pi - El_old;
    end
    
    if abs(Az_old) > FoV(1)/2 || abs(El_old) > FoV(2)/2
        Az(end-k) = 0.2*FoV(1)*(-1 + 2*rand(1,1));
        El(end-k) = 0.2*FoV(2)*(-1 + 2*rand(1,1));
        v_s = [cos(El(end-k))*cos(Az(end-k));...
            cos(El(end-k))*sin(Az(end-k));...
            sin(El(end-k))];
        A_err = [cos(psi)*cos(theta), cos(psi)*sin(theta)*sin(phi) + sin(psi)*cos(phi),...
            -cos(psi)*sin(theta)*cos(phi) + sin(psi)*sin(phi);...
            -sin(psi)*cos(theta), -sin(psi)*sin(theta)*sin(phi) + cos(psi)*cos(phi),...
            sin(psi)*sin(theta)*cos(phi) + cos(psi)*sin(phi);...
            sin(theta), -cos(theta)*sin(phi), cos(theta)*cos(phi)];
    else
        A_err = eye(3);
        v_s = v_s_old;
    end
   
   s_s = A_err*v_s;
   s_bTemp = A_bs*s_s;
   s_b(1:3, end-k) = s_bTemp./norm(s_bTemp); 
   v_nTemp = A_ns*v_s;
   v_n(1:3,end-k) = v_nTemp;
   v_n(1:3, end-k) = v_nTemp./norm(v_nTemp);
   
end

end

== matlab function library/Sensors/Light condition for the Sun sensor/Sun sensor/MATLAB Function ==
  data: phi input; A_err output; theta input; psi input
function A_err = error_matrix(phi, theta, psi)

A_err = [cos(psi)*cos(theta), cos(psi)*sin(theta)*sin(phi) + sin(psi)*cos(phi),...
    -cos(psi)*sin(theta)*cos(phi) + sin(psi)*sin(phi);...
    -sin(psi)*cos(theta), -sin(psi)*sin(theta)*sin(phi) + cos(psi)*cos(phi),...
    sin(psi)*sin(theta)*cos(phi) + cos(psi)*sin(phi);...
    sin(theta), -cos(theta)*sin(phi), cos(theta)*cos(phi)];
            
end

== matlab function library/Attitude determination/MATLAB Function ==
  data: s_b input; v_n input; sensors parameter; sunNotInFoV input; estQ output; q_old input
function estQ = QUEST(s_b, v_n, sensors, sunNotInFoV, q_old)

nM = size(s_b,2);

if sunNotInFoV
    a = (1/sensors.st.sigma)*ones(sensors.st.nStars, 1);
else
    a = [1/sensors.ss.sigma; (1/sensors.st.sigma)*ones(sensors.st.nStars - 1, 1)];
end

a = a./sum(a);
B = zeros(3);

for k = 1:nM
    B = B + a(k)*s_b(:,k)*v_n(:,k)';
end

z = [B(2,3) - B(3,2); B(3,1) - B(1,3); B(1,2) - B(2,1)];
sigma = trace(B);
S = B + B';

K = [S - sigma*eye(3), z;...
    z', sigma];

[V, lambdaMat] = eig(K);
lambda = diag(lambdaMat);
[~, idx] = max(lambda);
q = real(V(:,idx));

v = abs(q - q_old);
tol = 0.1*ones(4,1);

if sum(v > tol) ~= 0
    g = -1;
else
    g = 1;
end

estQ = g*q/norm(q);

end
